simulink model "Assegnamento_Autovalori"  (R2023b)
settings: Solver=VariableStepAuto  StartTime=0.0  StopTime=50  RelTol=1e-3
undefined symbols (not defined in the file): A, A_obs, B, B_obs, C, C_obs, D, D_obs, Ki, Kr
settings Model: Creator=emman  LastModifiedBy=emman

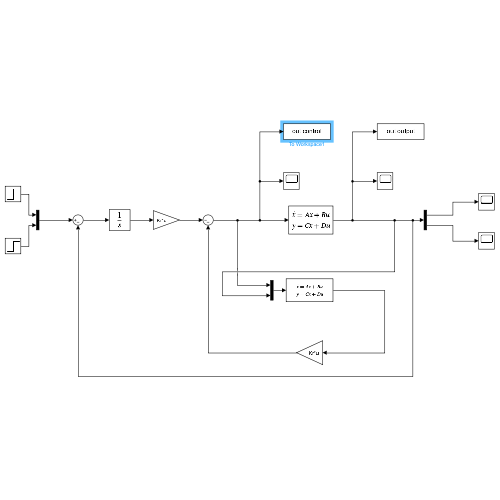
[thumbnail: Simulink's stored preview of the top-level diagram]
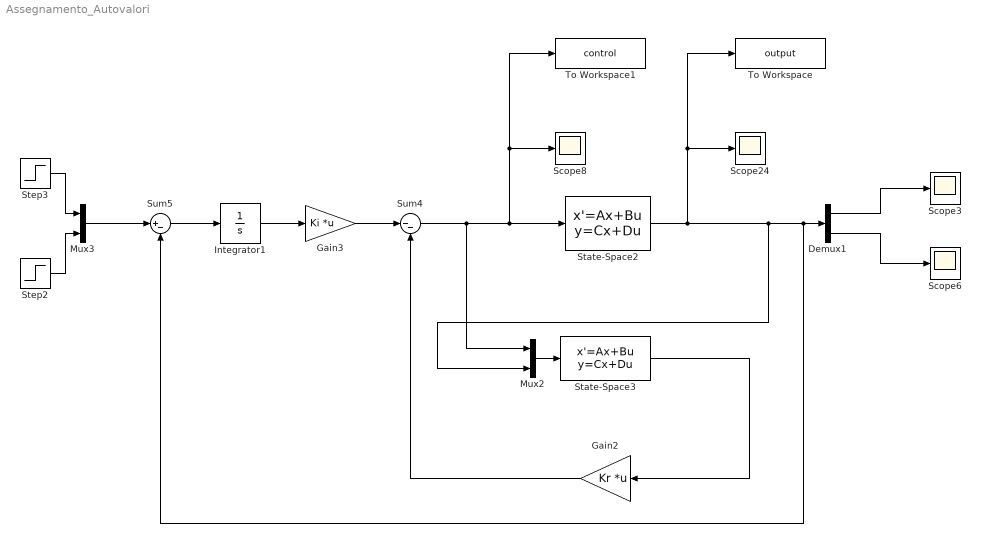
== system Assegnamento_Autovalori ==
  Demux1 : Demux  Outputs=2
  Gain2 : Gain  Gain=Kr  Multiplication=Matrix(K*u)
  Gain3 : Gain  Gain=Ki  Multiplication=Matrix(K*u)
  Integrator1 : Integrator
  Mux2 : Mux  Inputs=2
  Mux3 : Mux  Inputs=2
  Scope{3,6,8,24} (4 alike) : Scope
  State-Space2 : StateSpace  A=A  B=B  C=C  D=D  InitialCondition=0  ParameterTunability=Unconstrained
  State-Space3 : StateSpace  A=A_obs  B=B_obs  C=C_obs  D=D_obs  InitialCondition=0
  Step2 : Step  Time=0  After=2.5  SampleTime=0
  Step3 : Step  Time=0  After=2  SampleTime=0
  Sum4 : Sum  Inputs=|--
  Sum5 : Sum  Inputs=|+-
  To Workspace : ToWorkspace  VariableName=output  SaveFormat=Structure With Time  SampleTime=-1
  To Workspace1 : ToWorkspace  VariableName=control  SaveFormat=Structure With Time  SampleTime=-1
  wires:
  Demux1/1 -> Scope3/1
  Demux1/2 -> Scope6/1
  Integrator1/1 -> Gain3/1
  Gain3/1 -> Sum4/1
  Mux2/1 -> State-Space3/1
  Sum5/1 -> Integrator1/1
  State-Space3/1 -> Gain2/1
  Mux3/1 -> Sum5/1
  Step2/1 -> Mux3/2
  Gain2/1 -> Sum4/2
  Step3/1 -> Mux3/1
  State-Space2/1 -> To Workspace/1, Scope24/1, Sum5/2, Demux1/1, Mux2/2
  Sum4/1 -> To Workspace1/1, Scope8/1, State-Space2/1, Mux2/1
